simulink model "MASs_cp"  (R2015b)
settings: Solver=ode45  SolverMode=SingleTasking  StartTime=0.0  StopTime=10000  RelTol=1e-3
model workspace (MAT data in the model file):
  B = 3.17
  Cb = 0.251
  Izz = 1
  L = 9.8
  d = 0.71
  m = 5540
undefined symbols (not defined in the file or in its folder): magnitude
libraries: simulink x10
(part 1 of 2)
settings Model: Creator=Administrator  LastModifiedBy=Administrator
settings OptimizationCC: DefaultParameterBehavior=Inlined  UseFloatMulNetSlope=on  InlineInvariantSignals=on  PassReuseOutputArgsAs=Individual arguments  ZeroExternalMemoryAtStartup=off  ZeroInternalMemoryAtStartup=off  NoFixptDivByZeroProtection=on  EfficientFloat2IntCast=on  OptimizeModelRefInitCode=on  LifeSpan=1
settings HardwareCC: ProdBitPerPointer=32  ProdLargestAtomicInteger=Long  ProdLargestAtomicFloat=Double  ProdWordSize=32  ProdHWDeviceType=NXP->Cortex-M4
settings RTWCC: SystemTargetFile=ert.tlc  TemplateMakefile=ert_default_tmf  Description=Embedded Coder  GenerateReport=on  IncludeHyperlinkInReport=on  LaunchReport=on  GenerateTraceInfo=on  GenerateTraceReport=on  GenerateTraceReportSl=on  GenerateTraceReportSf=on  GenerateTraceReportEml=on  GenerateCodeMetricsReport=on
settings CodeAppCC: ForceParamTrailComments=on  IgnoreCustomStorageClasses=off  SimulinkDataObjDesc=on  CustomSymbolStrGlobalVar=rt$N$M  CustomSymbolStrType=$N$M  CustomSymbolStrFcn=$N$M$F  CustomSymbolStrMacro=$N$M  InsertBlockDesc=on
settings ERTTargetCC: GenerateSampleERTMain=on  IncludeMdlTerminateFcn=off  CombineSignalStateStructs=on  SupportNonFinite=off  SupportContinuousTime=on  InlinedParameterPlacement=NonHierarchical  ERTCustomFileTemplate=example_file_process.tlc  ERTFilePackagingFormat=CompactWithDataFile

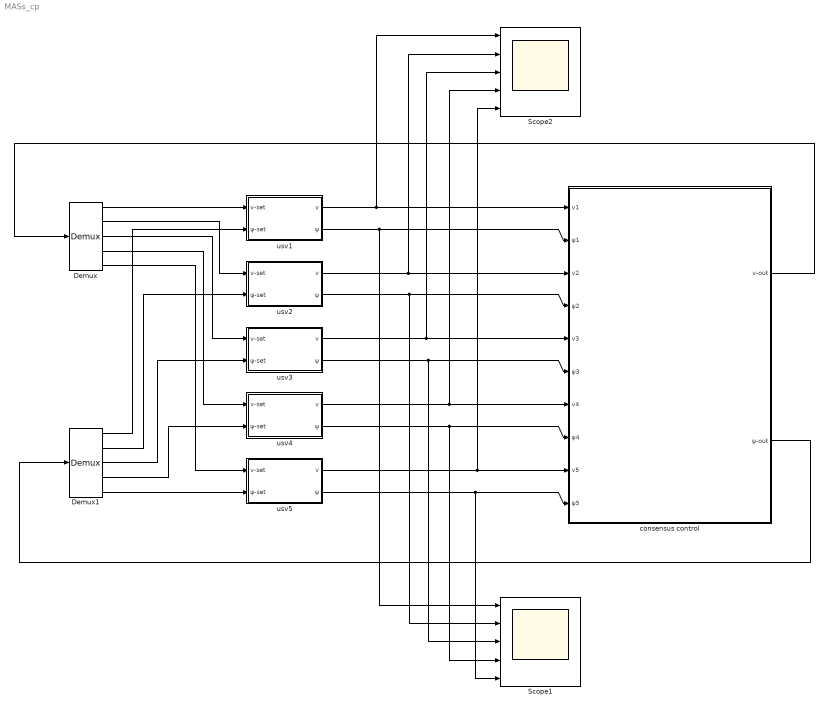
== system MASs_cp ==
  Demux : Demux  Outputs=5
  Demux1 : Demux  Outputs=5
  Scope1 : Scope  NumInputPorts=5
  Scope2 : Scope  NumInputPorts=5
  consensus control : Subsystem
  usv1 : Subsystem
  usv2 : Subsystem
  usv3 : Subsystem
  usv4 : Subsystem
  usv5 : Subsystem
  wires:
  usv1/2(ψ) -> Scope1/1, consensus control/2(ψ1)
  usv2/2(ψ) -> Scope1/2, consensus control/4(ψ2)
  usv3/2(ψ) -> Scope1/3, consensus control/6(ψ3)
  usv4/2(ψ) -> Scope1/4, consensus control/8(ψ4)
  usv5/2(ψ) -> Scope1/5, consensus control/10(ψ5)
  Demux/1 -> usv1/1(v-set)
  Demux/2 -> usv2/1(v-set)
  Demux/3 -> usv3/1(v-set)
  Demux/4 -> usv4/1(v-set)
  Demux/5 -> usv5/1(v-set)
  Demux1/2 -> usv2/2(ψ-set)
  Demux1/3 -> usv3/2(ψ-set)
  Demux1/4 -> usv4/2(ψ-set)
  Demux1/5 -> usv5/2(ψ-set)
  Demux1/1 -> usv1/2(ψ-set)
  usv1/1(v) -> Scope2/1, consensus control/1(v1)
  usv2/1(v) -> Scope2/2, consensus control/3(v2)
  usv3/1(v) -> Scope2/3, consensus control/5(v3)
  usv4/1(v) -> Scope2/4, consensus control/7(v4)
  usv5/1(v) -> Scope2/5, consensus control/9(v5)
  consensus control/2(ψ-out) -> Demux1/1
  consensus control/1(v-out) -> Demux/1

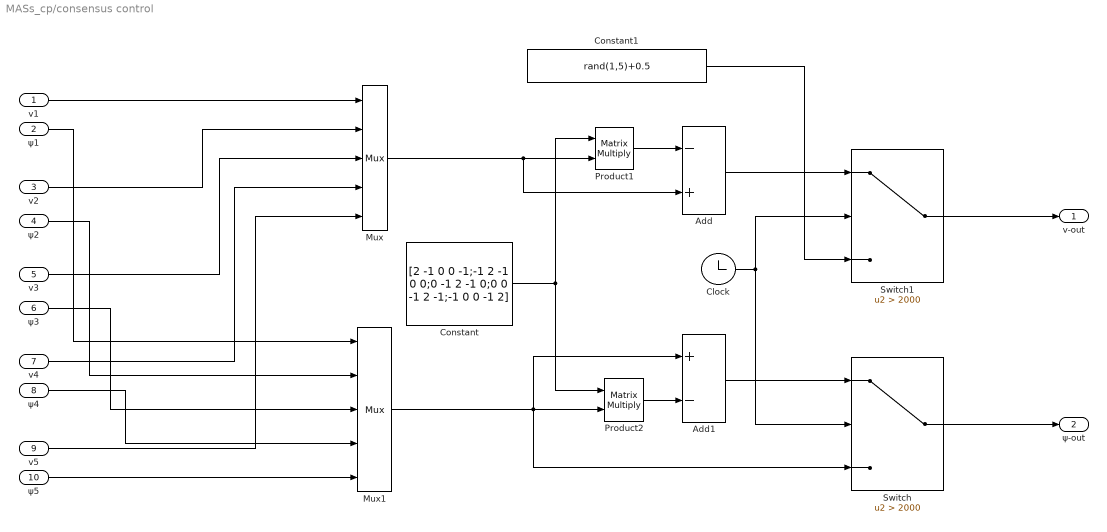
== system MASs_cp/consensus control ==
  v1 : Inport
  ψ1 : Inport  Port=2
  v2 : Inport  Port=3
  ψ2 : Inport  Port=4
  v3 : Inport  Port=5
  ψ3 : Inport  Port=6
  v4 : Inport  Port=7
  ψ4 : Inport  Port=8
  v5 : Inport  Port=9
  ψ5 : Inport  Port=10
  Add : Sum  Inputs=-+
  Add1 : Sum  Inputs=+-
  Clock : Clock
  Constant : Constant  Value=[2 -1 0 0 -1;-1 2 -1 0 0;0 -1 2 -1 0;0 0 -1 2 -1;-1 0 0 -1 2]  VectorParams1D=off
  Constant1 : Constant  Value=rand(1,5)+0.5
  Mux : Mux  Inputs=5
  Mux1 : Mux  Inputs=5
  Product1 : Product  Multiplication=Matrix(*)
  Product2 : Product  Multiplication=Matrix(*)
  Switch : Switch  Criteria=u2 > Threshold  Threshold=2000
  Switch1 : Switch  Criteria=u2 > Threshold  Threshold=2000
  v-out : Outport
  ψ-out : Outport  Port=2
  wires:
  Mux/1 -> Add/2, Product1/2
  Add/1 -> Switch1/1
  Product1/1 -> Add/1
  v4/1 -> Mux/4
  v5/1 -> Mux/5
  Mux1/1 -> Switch/3, Add1/1, Product2/2
  Product2/1 -> Add1/2
  ψ4/1 -> Mux1/4
  ψ1/1 -> Mux1/1
  ψ2/1 -> Mux1/2
  ψ3/1 -> Mux1/3
  ψ5/1 -> Mux1/5
  Add1/1 -> Switch/1
  v3/1 -> Mux/3
  v2/1 -> Mux/2
  Constant/1 -> Product2/1, Product1/1
  v1/1 -> Mux/1
  Clock/1 -> Switch/2, Switch1/2
  Switch/1 -> ψ-out/1
  Constant1/1 -> Switch1/3
  Switch1/1 -> v-out/1

== system MASs_cp/usv1 ==
  v-set : Inport
  ψ-set : Inport  Port=2
  Scope : Scope  NumInputPorts=3
  Scope1 : Scope  NumInputPorts=3
  To Workspace : ToWorkspace  VariableName=x1  SampleTime=-1
  To Workspace1 : ToWorkspace  VariableName=y1  SampleTime=-1
  USV : Subsystem
  direction-PID : Subsystem
  speed-PID : Subsystem
  v : Outport
  ψ : Outport  Port=2
  wires:
  speed-PID/1(output) -> USV/1(n)
  USV/6(ψ) -> Scope1/3, ψ/1, direction-PID/2(feedback)
  USV/3(r) -> Scope/3
  direction-PID/1(output) -> USV/2(δ)
  v-set/1 -> speed-PID/2(set)
  USV/2(v) -> Scope/2
  ψ-set/1 -> direction-PID/1(set)
  USV/5(y) -> To Workspace1/1, Scope1/2
  USV/4(x) -> To Workspace/1, Scope1/1
  USV/1(u) -> v/1, speed-PID/1(feedback), Scope/1

== system MASs_cp/usv2 ==
  v-set : Inport
  ψ-set : Inport  Port=2
  Scope : Scope  NumInputPorts=3
  Scope1 : Scope  NumInputPorts=3
  To Workspace : ToWorkspace  VariableName=x2  SampleTime=-1
  To Workspace1 : ToWorkspace  VariableName=y2  SampleTime=-1
  USV : Subsystem
  direction-PID : Subsystem
  speed-PID : Subsystem
  v : Outport
  ψ : Outport  Port=2
  wires:
  speed-PID/1(output) -> USV/1(n)
  USV/6(ψ) -> Scope1/3, ψ/1, direction-PID/2(feedback)
  USV/3(r) -> Scope/3
  direction-PID/1(output) -> USV/2(δ)
  v-set/1 -> speed-PID/2(set)
  USV/2(v) -> Scope/2
  ψ-set/1 -> direction-PID/1(set)
  USV/5(y) -> To Workspace1/1, Scope1/2
  USV/4(x) -> To Workspace/1, Scope1/1
  USV/1(u) -> speed-PID/1(feedback), v/1, Scope/1

== system MASs_cp/usv3 ==
  v-set : Inport
  ψ-set : Inport  Port=2
  Scope : Scope  NumInputPorts=3
  Scope1 : Scope  NumInputPorts=3
  To Workspace : ToWorkspace  VariableName=x3  SampleTime=-1
  To Workspace1 : ToWorkspace  VariableName=y3  SampleTime=-1
  USV : Subsystem
  direction-PID1 : Subsystem
  speed-PID : Subsystem
  v : Outport
  ψ : Outport  Port=2
  wires:
  speed-PID/1(output) -> USV/1(n)
  USV/6(ψ) -> Scope1/3, direction-PID1/2(feedback), ψ/1
  USV/3(r) -> Scope/3
  direction-PID1/1(output) -> USV/2(δ)
  v-set/1 -> speed-PID/2(set)
  USV/2(v) -> Scope/2
  ψ-set/1 -> direction-PID1/1(set)
  USV/5(y) -> To Workspace1/1, Scope1/2
  USV/4(x) -> To Workspace/1, Scope1/1
  USV/1(u) -> speed-PID/1(feedback), v/1, Scope/1

== system MASs_cp/usv4 ==
  v-set : Inport
  ψ-set : Inport  Port=2
  Scope : Scope  NumInputPorts=3
  Scope1 : Scope  NumInputPorts=3
  To Workspace : ToWorkspace  VariableName=x4  SampleTime=-1
  To Workspace1 : ToWorkspace  VariableName=y4  SampleTime=-1
  USV : Subsystem
  direction-PID : Subsystem
  speed-PID : Subsystem
  v : Outport
  ψ : Outport  Port=2
  wires:
  speed-PID/1(output) -> USV/1(n)
  USV/6(ψ) -> Scope1/3, direction-PID/2(feedback), ψ/1
  USV/3(r) -> Scope/3
  direction-PID/1(output) -> USV/2(δ)
  v-set/1 -> speed-PID/2(set)
  USV/2(v) -> Scope/2
  ψ-set/1 -> direction-PID/1(set)
  USV/5(y) -> To Workspace1/1, Scope1/2
  USV/4(x) -> To Workspace/1, Scope1/1
  USV/1(u) -> speed-PID/1(feedback), v/1, Scope/1

== system MASs_cp/usv5 ==
  v-set : Inport
  ψ-set : Inport  Port=2
  Scope : Scope  NumInputPorts=3
  Scope1 : Scope  NumInputPorts=3
  To Workspace : ToWorkspace  VariableName=x5  SampleTime=-1
  To Workspace1 : ToWorkspace  VariableName=y5  SampleTime=-1
  USV : Subsystem
  direction-PID : Subsystem
  speed-PID : Subsystem
  v : Outport
  ψ : Outport  Port=2
  wires:
  speed-PID/1(output) -> USV/1(n)
  USV/6(ψ) -> Scope1/3, direction-PID/2(feedback), ψ/1
  USV/3(r) -> Scope/3
  direction-PID/1(output) -> USV/2(δ)
  v-set/1 -> speed-PID/2(set)
  USV/2(v) -> Scope/2
  ψ-set/1 -> direction-PID/1(set)
  USV/5(y) -> To Workspace1/1, Scope1/2
  USV/4(x) -> To Workspace/1, Scope1/1
  USV/1(u) -> speed-PID/1(feedback), v/1, Scope/1

== system MASs_cp/usv1/USV ==
  n : Inport
  δ : Inport  Port=2
  F model : Subsystem
  M model : Subsystem
  motion model : Subsystem
  u : Outport
  v : Outport  Port=2
  r : Outport  Port=3
  x : Outport  Port=4
  y : Outport  Port=5
  ψ : Outport  Port=6
  wires:
  M model/5(Jzz) -> motion model/8(Jzz)
  M model/3(my) -> motion model/6(my)
  M model/1(m) -> motion model/4(m)
  F model/2(Y) -> motion model/2(Y)
  n/1 -> F model/1(n)
  δ/1 -> F model/2(δ)
  F model/1(X) -> motion model/1(X)
  motion model/1(u) -> u/1, F model/3(u)  "u"
  motion model/3(r) -> r/1, F model/5(r)  "r"
  motion model/2(v) -> v/1, F model/4(v)  "v"
  motion model/6(ψ) -> ψ/1  "ψ"
  F model/3(N) -> motion model/3(N)
  M model/2(mx) -> motion model/5(mx)
  M model/4(Izz) -> motion model/7(Izz)
  motion model/4(x) -> x/1  "x"
  motion model/5(y) -> y/1  "y"

== system MASs_cp/usv1/direction-PID ==
  set : Inport
  feedback : Inport  Port=2
  Gain : Gain  Gain=-1
  PID Controller : simulink/Continuous/PID Controller  Controller=PID  TimeDomain=Continuous-time  SampleTime=-1  IntegratorMethod=Forward Euler  FilterMethod=Forward Euler  Form=Parallel  UseFilter=on  ControllerParametersSource=internal  P=3  I=0  D=0  N=5.45397025421619  InitialConditionSource=internal  InitialConditionForIntegrator=0  InitialConditionForFilter=0  ExternalReset=none  LimitOutput=on  UpperSaturationLimit=50  LowerSaturationLimit=-50  LinearizeAsGain=on  AntiWindupMode=none  Kb=1  TrackingMode=off  Kt=1  PParamMin=[]  PParamMax=[]  IParamMin=[]  IParamMax=[]  DParamMin=[]  DParamMax=[]  NParamMin=[]  NParamMax=[]  KbParamMin=[]  KbParamMax=[]  KtParamMin=[]  KtParamMax=[]  POutMin=[]  POutMax=[]  IOutMin=[]  IOutMax=[]  DOutMin=[]  DOutMax=[]  NOutMin=[]  NOutMax=[]  KbOutMin=[]  KbOutMax=[]  KtOutMin=[]  KtOutMax=[]  IntegratorOutMin=[]  IntegratorOutMax=[]  FilterOutMin=[]  FilterOutMax=[]  SumOutMin=[]  SumOutMax=[]  SumI1OutMin=[]  SumI1OutMax=[]  SumI2OutMin=[]  SumI2OutMax=[]  SumI3OutMin=[]  SumI3OutMax=[]  SumDOutMin=[]  SumDOutMax=[]  SaturationOutMin=[]  SaturationOutMax=[]  IntegratorContinuousStateAttributes=''  IntegratorStateMustResolveToSignalObject=off  IntegratorRTWStateStorageClass=Auto  FilterContinuousStateAttributes=''  FilterStateMustResolveToSignalObject=off  FilterRTWStateStorageClass=Auto  DifferentiatorICPrevScaledInput=0  DifferentiatorOutMin=[]  DifferentiatorOutMax=[]
  Scope2 : Scope  NumInputPorts=3
  Sum : Sum  Inputs=|+-
  output : Outport
  wires:
  PID Controller/1 -> Gain/1, Scope2/3
  Sum/1 -> PID Controller/1
  set/1 -> Scope2/1, Sum/1
  feedback/1 -> Scope2/2, Sum/2
  Gain/1 -> output/1

== system MASs_cp/usv1/speed-PID ==
  feedback : Inport
  set : Inport  Port=2
  PID Controller : simulink/Continuous/PID Controller  Controller=PID  TimeDomain=Continuous-time  SampleTime=-1  IntegratorMethod=Forward Euler  FilterMethod=Forward Euler  Form=Parallel  UseFilter=on  ControllerParametersSource=internal  P=500  I=2  D=0  N=5.45397025421619  InitialConditionSource=internal  InitialConditionForIntegrator=0  InitialConditionForFilter=0  ExternalReset=none  LimitOutput=on  UpperSaturationLimit=2000  LowerSaturationLimit=0  LinearizeAsGain=on  AntiWindupMode=none  Kb=1  TrackingMode=off  Kt=1  PParamMin=[]  PParamMax=[]  IParamMin=[]  IParamMax=[]  DParamMin=[]  DParamMax=[]  NParamMin=[]  NParamMax=[]  KbParamMin=[]  KbParamMax=[]  KtParamMin=[]  KtParamMax=[]  POutMin=[]  POutMax=[]  IOutMin=[]  IOutMax=[]  DOutMin=[]  DOutMax=[]  NOutMin=[]  NOutMax=[]  KbOutMin=[]  KbOutMax=[]  KtOutMin=[]  KtOutMax=[]  IntegratorOutMin=[]  IntegratorOutMax=[]  FilterOutMin=[]  FilterOutMax=[]  SumOutMin=[]  SumOutMax=[]  SumI1OutMin=[]  SumI1OutMax=[]  SumI2OutMin=[]  SumI2OutMax=[]  SumI3OutMin=[]  SumI3OutMax=[]  SumDOutMin=[]  SumDOutMax=[]  SaturationOutMin=[]  SaturationOutMax=[]  IntegratorContinuousStateAttributes=''  IntegratorStateMustResolveToSignalObject=off  IntegratorRTWStateStorageClass=Auto  FilterContinuousStateAttributes=''  FilterStateMustResolveToSignalObject=off  FilterRTWStateStorageClass=Auto  DifferentiatorICPrevScaledInput=0  DifferentiatorOutMin=[]  DifferentiatorOutMax=[]
  Scope3 : Scope  NumInputPorts=3
  Sum1 : Sum  Inputs=|+-
  output : Outport
  wires:
  set/1 -> Sum1/1, Scope3/1
  PID Controller/1 -> output/1, Scope3/3
  Sum1/1 -> PID Controller/1
  feedback/1 -> Sum1/2, Scope3/2

== system MASs_cp/usv2/USV ==
  n : Inport
  δ : Inport  Port=2
  F model : Subsystem
  M model : Subsystem
  motion model : Subsystem
  u : Outport
  v : Outport  Port=2
  r : Outport  Port=3
  x : Outport  Port=4
  y : Outport  Port=5
  ψ : Outport  Port=6
  wires:
  M model/5(Jzz) -> motion model/8(Jzz)
  M model/3(my) -> motion model/6(my)
  M model/1(m) -> motion model/4(m)
  F model/2(Y) -> motion model/2(Y)
  n/1 -> F model/1(n)
  δ/1 -> F model/2(δ)
  F model/1(X) -> motion model/1(X)
  motion model/1(u) -> u/1, F model/3(u)  "u"
  motion model/3(r) -> r/1, F model/5(r)  "r"
  motion model/2(v) -> v/1, F model/4(v)  "v"
  motion model/6(ψ) -> ψ/1  "ψ"
  F model/3(N) -> motion model/3(N)
  M model/2(mx) -> motion model/5(mx)
  M model/4(Izz) -> motion model/7(Izz)
  motion model/4(x) -> x/1  "x"
  motion model/5(y) -> y/1  "y"

== system MASs_cp/usv2/direction-PID ==
  set : Inport
  feedback : Inport  Port=2
  Gain : Gain  Gain=-1
  PID Controller : simulink/Continuous/PID Controller  Controller=PID  TimeDomain=Continuous-time  SampleTime=-1  IntegratorMethod=Forward Euler  FilterMethod=Forward Euler  Form=Parallel  UseFilter=on  ControllerParametersSource=internal  P=3  I=0  D=0  N=5.45397025421619  InitialConditionSource=internal  InitialConditionForIntegrator=0  InitialConditionForFilter=0  ExternalReset=none  LimitOutput=on  UpperSaturationLimit=50  LowerSaturationLimit=-50  LinearizeAsGain=on  AntiWindupMode=none  Kb=1  TrackingMode=off  Kt=1  PParamMin=[]  PParamMax=[]  IParamMin=[]  IParamMax=[]  DParamMin=[]  DParamMax=[]  NParamMin=[]  NParamMax=[]  KbParamMin=[]  KbParamMax=[]  KtParamMin=[]  KtParamMax=[]  POutMin=[]  POutMax=[]  IOutMin=[]  IOutMax=[]  DOutMin=[]  DOutMax=[]  NOutMin=[]  NOutMax=[]  KbOutMin=[]  KbOutMax=[]  KtOutMin=[]  KtOutMax=[]  IntegratorOutMin=[]  IntegratorOutMax=[]  FilterOutMin=[]  FilterOutMax=[]  SumOutMin=[]  SumOutMax=[]  SumI1OutMin=[]  SumI1OutMax=[]  SumI2OutMin=[]  SumI2OutMax=[]  SumI3OutMin=[]  SumI3OutMax=[]  SumDOutMin=[]  SumDOutMax=[]  SaturationOutMin=[]  SaturationOutMax=[]  IntegratorContinuousStateAttributes=''  IntegratorStateMustResolveToSignalObject=off  IntegratorRTWStateStorageClass=Auto  FilterContinuousStateAttributes=''  FilterStateMustResolveToSignalObject=off  FilterRTWStateStorageClass=Auto  DifferentiatorICPrevScaledInput=0  DifferentiatorOutMin=[]  DifferentiatorOutMax=[]
  Scope2 : Scope  NumInputPorts=3
  Sum : Sum  Inputs=|+-
  output : Outport
  wires:
  PID Controller/1 -> Gain/1, Scope2/3
  Sum/1 -> PID Controller/1
  set/1 -> Scope2/1, Sum/1
  feedback/1 -> Scope2/2, Sum/2
  Gain/1 -> output/1

== system MASs_cp/usv2/speed-PID ==
  feedback : Inport
  set : Inport  Port=2
  PID Controller : simulink/Continuous/PID Controller  Controller=PID  TimeDomain=Continuous-time  SampleTime=-1  IntegratorMethod=Forward Euler  FilterMethod=Forward Euler  Form=Parallel  UseFilter=on  ControllerParametersSource=internal  P=500  I=2  D=0  N=5.45397025421619  InitialConditionSource=internal  InitialConditionForIntegrator=0  InitialConditionForFilter=0  ExternalReset=none  LimitOutput=on  UpperSaturationLimit=2000  LowerSaturationLimit=0  LinearizeAsGain=on  AntiWindupMode=none  Kb=1  TrackingMode=off  Kt=1  PParamMin=[]  PParamMax=[]  IParamMin=[]  IParamMax=[]  DParamMin=[]  DParamMax=[]  NParamMin=[]  NParamMax=[]  KbParamMin=[]  KbParamMax=[]  KtParamMin=[]  KtParamMax=[]  POutMin=[]  POutMax=[]  IOutMin=[]  IOutMax=[]  DOutMin=[]  DOutMax=[]  NOutMin=[]  NOutMax=[]  KbOutMin=[]  KbOutMax=[]  KtOutMin=[]  KtOutMax=[]  IntegratorOutMin=[]  IntegratorOutMax=[]  FilterOutMin=[]  FilterOutMax=[]  SumOutMin=[]  SumOutMax=[]  SumI1OutMin=[]  SumI1OutMax=[]  SumI2OutMin=[]  SumI2OutMax=[]  SumI3OutMin=[]  SumI3OutMax=[]  SumDOutMin=[]  SumDOutMax=[]  SaturationOutMin=[]  SaturationOutMax=[]  IntegratorContinuousStateAttributes=''  IntegratorStateMustResolveToSignalObject=off  IntegratorRTWStateStorageClass=Auto  FilterContinuousStateAttributes=''  FilterStateMustResolveToSignalObject=off  FilterRTWStateStorageClass=Auto  DifferentiatorICPrevScaledInput=0  DifferentiatorOutMin=[]  DifferentiatorOutMax=[]
  Scope3 : Scope  NumInputPorts=3
  Sum1 : Sum  Inputs=|+-
  output : Outport
  wires:
  set/1 -> Sum1/1, Scope3/1
  PID Controller/1 -> output/1, Scope3/3
  Sum1/1 -> PID Controller/1
  feedback/1 -> Sum1/2, Scope3/2

== system MASs_cp/usv3/USV ==
  n : Inport
  δ : Inport  Port=2
  F model : Subsystem
  M model : Subsystem
  motion model : Subsystem
  u : Outport
  v : Outport  Port=2
  r : Outport  Port=3
  x : Outport  Port=4
  y : Outport  Port=5
  ψ : Outport  Port=6
  wires:
  M model/5(Jzz) -> motion model/8(Jzz)
  M model/3(my) -> motion model/6(my)
  M model/1(m) -> motion model/4(m)
  F model/2(Y) -> motion model/2(Y)
  n/1 -> F model/1(n)
  δ/1 -> F model/2(δ)
  F model/1(X) -> motion model/1(X)
  motion model/1(u) -> u/1, F model/3(u)  "u"
  motion model/3(r) -> r/1, F model/5(r)  "r"
  motion model/2(v) -> v/1, F model/4(v)  "v"
  motion model/6(ψ) -> ψ/1  "ψ"
  F model/3(N) -> motion model/3(N)
  M model/2(mx) -> motion model/5(mx)
  M model/4(Izz) -> motion model/7(Izz)
  motion model/4(x) -> x/1  "x"
  motion model/5(y) -> y/1  "y"

== system MASs_cp/usv3/direction-PID1 ==
  set : Inport
  feedback : Inport  Port=2
  Gain : Gain  Gain=-1
  PID Controller : simulink/Continuous/PID Controller  Controller=PID  TimeDomain=Continuous-time  SampleTime=-1  IntegratorMethod=Forward Euler  FilterMethod=Forward Euler  Form=Parallel  UseFilter=on  ControllerParametersSource=internal  P=3  I=0  D=0  N=5.45397025421619  InitialConditionSource=internal  InitialConditionForIntegrator=0  InitialConditionForFilter=0  ExternalReset=none  LimitOutput=on  UpperSaturationLimit=50  LowerSaturationLimit=-50  LinearizeAsGain=on  AntiWindupMode=none  Kb=1  TrackingMode=off  Kt=1  PParamMin=[]  PParamMax=[]  IParamMin=[]  IParamMax=[]  DParamMin=[]  DParamMax=[]  NParamMin=[]  NParamMax=[]  KbParamMin=[]  KbParamMax=[]  KtParamMin=[]  KtParamMax=[]  POutMin=[]  POutMax=[]  IOutMin=[]  IOutMax=[]  DOutMin=[]  DOutMax=[]  NOutMin=[]  NOutMax=[]  KbOutMin=[]  KbOutMax=[]  KtOutMin=[]  KtOutMax=[]  IntegratorOutMin=[]  IntegratorOutMax=[]  FilterOutMin=[]  FilterOutMax=[]  SumOutMin=[]  SumOutMax=[]  SumI1OutMin=[]  SumI1OutMax=[]  SumI2OutMin=[]  SumI2OutMax=[]  SumI3OutMin=[]  SumI3OutMax=[]  SumDOutMin=[]  SumDOutMax=[]  SaturationOutMin=[]  SaturationOutMax=[]  IntegratorContinuousStateAttributes=''  IntegratorStateMustResolveToSignalObject=off  IntegratorRTWStateStorageClass=Auto  FilterContinuousStateAttributes=''  FilterStateMustResolveToSignalObject=off  FilterRTWStateStorageClass=Auto  DifferentiatorICPrevScaledInput=0  DifferentiatorOutMin=[]  DifferentiatorOutMax=[]
  Scope2 : Scope  NumInputPorts=3
  Sum : Sum  Inputs=|+-
  output : Outport
  wires:
  PID Controller/1 -> Gain/1, Scope2/3
  Sum/1 -> PID Controller/1
  set/1 -> Scope2/1, Sum/1
  feedback/1 -> Scope2/2, Sum/2
  Gain/1 -> output/1

== system MASs_cp/usv3/speed-PID ==
  feedback : Inport
  set : Inport  Port=2
  PID Controller : simulink/Continuous/PID Controller  Controller=PID  TimeDomain=Continuous-time  SampleTime=-1  IntegratorMethod=Forward Euler  FilterMethod=Forward Euler  Form=Parallel  UseFilter=on  ControllerParametersSource=internal  P=500  I=2  D=0  N=5.45397025421619  InitialConditionSource=internal  InitialConditionForIntegrator=0  InitialConditionForFilter=0  ExternalReset=none  LimitOutput=on  UpperSaturationLimit=2000  LowerSaturationLimit=0  LinearizeAsGain=on  AntiWindupMode=none  Kb=1  TrackingMode=off  Kt=1  PParamMin=[]  PParamMax=[]  IParamMin=[]  IParamMax=[]  DParamMin=[]  DParamMax=[]  NParamMin=[]  NParamMax=[]  KbParamMin=[]  KbParamMax=[]  KtParamMin=[]  KtParamMax=[]  POutMin=[]  POutMax=[]  IOutMin=[]  IOutMax=[]  DOutMin=[]  DOutMax=[]  NOutMin=[]  NOutMax=[]  KbOutMin=[]  KbOutMax=[]  KtOutMin=[]  KtOutMax=[]  IntegratorOutMin=[]  IntegratorOutMax=[]  FilterOutMin=[]  FilterOutMax=[]  SumOutMin=[]  SumOutMax=[]  SumI1OutMin=[]  SumI1OutMax=[]  SumI2OutMin=[]  SumI2OutMax=[]  SumI3OutMin=[]  SumI3OutMax=[]  SumDOutMin=[]  SumDOutMax=[]  SaturationOutMin=[]  SaturationOutMax=[]  IntegratorContinuousStateAttributes=''  IntegratorStateMustResolveToSignalObject=off  IntegratorRTWStateStorageClass=Auto  FilterContinuousStateAttributes=''  FilterStateMustResolveToSignalObject=off  FilterRTWStateStorageClass=Auto  DifferentiatorICPrevScaledInput=0  DifferentiatorOutMin=[]  DifferentiatorOutMax=[]
  Scope3 : Scope  NumInputPorts=3
  Sum1 : Sum  Inputs=|+-
  output : Outport
  wires:
  set/1 -> Sum1/1, Scope3/1
  PID Controller/1 -> output/1, Scope3/3
  Sum1/1 -> PID Controller/1
  feedback/1 -> Sum1/2, Scope3/2

== system MASs_cp/usv4/USV ==
  n : Inport
  δ : Inport  Port=2
  F model : Subsystem
  M model : Subsystem
  motion model : Subsystem
  u : Outport
  v : Outport  Port=2
  r : Outport  Port=3
  x : Outport  Port=4
  y : Outport  Port=5
  ψ : Outport  Port=6
  wires:
  M model/5(Jzz) -> motion model/8(Jzz)
  M model/3(my) -> motion model/6(my)
  M model/1(m) -> motion model/4(m)
  F model/2(Y) -> motion model/2(Y)
  n/1 -> F model/1(n)
  δ/1 -> F model/2(δ)
  F model/1(X) -> motion model/1(X)
  motion model/1(u) -> u/1, F model/3(u)  "u"
  motion model/3(r) -> r/1, F model/5(r)  "r"
  motion model/2(v) -> v/1, F model/4(v)  "v"
  motion model/6(ψ) -> ψ/1  "ψ"
  F model/3(N) -> motion model/3(N)
  M model/2(mx) -> motion model/5(mx)
  M model/4(Izz) -> motion model/7(Izz)
  motion model/4(x) -> x/1  "x"
  motion model/5(y) -> y/1  "y"

== system MASs_cp/usv4/direction-PID ==
  set : Inport
  feedback : Inport  Port=2
  Gain : Gain  Gain=-1
  PID Controller : simulink/Continuous/PID Controller  Controller=PID  TimeDomain=Continuous-time  SampleTime=-1  IntegratorMethod=Forward Euler  FilterMethod=Forward Euler  Form=Parallel  UseFilter=on  ControllerParametersSource=internal  P=3  I=0  D=0  N=5.45397025421619  InitialConditionSource=internal  InitialConditionForIntegrator=0  InitialConditionForFilter=0  ExternalReset=none  LimitOutput=on  UpperSaturationLimit=50  LowerSaturationLimit=-50  LinearizeAsGain=on  AntiWindupMode=none  Kb=1  TrackingMode=off  Kt=1  PParamMin=[]  PParamMax=[]  IParamMin=[]  IParamMax=[]  DParamMin=[]  DParamMax=[]  NParamMin=[]  NParamMax=[]  KbParamMin=[]  KbParamMax=[]  KtParamMin=[]  KtParamMax=[]  POutMin=[]  POutMax=[]  IOutMin=[]  IOutMax=[]  DOutMin=[]  DOutMax=[]  NOutMin=[]  NOutMax=[]  KbOutMin=[]  KbOutMax=[]  KtOutMin=[]  KtOutMax=[]  IntegratorOutMin=[]  IntegratorOutMax=[]  FilterOutMin=[]  FilterOutMax=[]  SumOutMin=[]  SumOutMax=[]  SumI1OutMin=[]  SumI1OutMax=[]  SumI2OutMin=[]  SumI2OutMax=[]  SumI3OutMin=[]  SumI3OutMax=[]  SumDOutMin=[]  SumDOutMax=[]  SaturationOutMin=[]  SaturationOutMax=[]  IntegratorContinuousStateAttributes=''  IntegratorStateMustResolveToSignalObject=off  IntegratorRTWStateStorageClass=Auto  FilterContinuousStateAttributes=''  FilterStateMustResolveToSignalObject=off  FilterRTWStateStorageClass=Auto  DifferentiatorICPrevScaledInput=0  DifferentiatorOutMin=[]  DifferentiatorOutMax=[]
  Scope2 : Scope  NumInputPorts=3
  Sum : Sum  Inputs=|+-
  output : Outport
  wires:
  PID Controller/1 -> Gain/1, Scope2/3
  Sum/1 -> PID Controller/1
  set/1 -> Scope2/1, Sum/1
  feedback/1 -> Scope2/2, Sum/2
  Gain/1 -> output/1

== system MASs_cp/usv4/speed-PID ==
  feedback : Inport
  set : Inport  Port=2
  PID Controller : simulink/Continuous/PID Controller  Controller=PID  TimeDomain=Continuous-time  SampleTime=-1  IntegratorMethod=Forward Euler  FilterMethod=Forward Euler  Form=Parallel  UseFilter=on  ControllerParametersSource=internal  P=500  I=2  D=0  N=5.45397025421619  InitialConditionSource=internal  InitialConditionForIntegrator=0  InitialConditionForFilter=0  ExternalReset=none  LimitOutput=on  UpperSaturationLimit=2000  LowerSaturationLimit=0  LinearizeAsGain=on  AntiWindupMode=none  Kb=1  TrackingMode=off  Kt=1  PParamMin=[]  PParamMax=[]  IParamMin=[]  IParamMax=[]  DParamMin=[]  DParamMax=[]  NParamMin=[]  NParamMax=[]  KbParamMin=[]  KbParamMax=[]  KtParamMin=[]  KtParamMax=[]  POutMin=[]  POutMax=[]  IOutMin=[]  IOutMax=[]  DOutMin=[]  DOutMax=[]  NOutMin=[]  NOutMax=[]  KbOutMin=[]  KbOutMax=[]  KtOutMin=[]  KtOutMax=[]  IntegratorOutMin=[]  IntegratorOutMax=[]  FilterOutMin=[]  FilterOutMax=[]  SumOutMin=[]  SumOutMax=[]  SumI1OutMin=[]  SumI1OutMax=[]  SumI2OutMin=[]  SumI2OutMax=[]  SumI3OutMin=[]  SumI3OutMax=[]  SumDOutMin=[]  SumDOutMax=[]  SaturationOutMin=[]  SaturationOutMax=[]  IntegratorContinuousStateAttributes=''  IntegratorStateMustResolveToSignalObject=off  IntegratorRTWStateStorageClass=Auto  FilterContinuousStateAttributes=''  FilterStateMustResolveToSignalObject=off  FilterRTWStateStorageClass=Auto  DifferentiatorICPrevScaledInput=0  DifferentiatorOutMin=[]  DifferentiatorOutMax=[]
  Scope3 : Scope  NumInputPorts=3
  Sum1 : Sum  Inputs=|+-
  output : Outport
  wires:
  set/1 -> Sum1/1, Scope3/1
  PID Controller/1 -> output/1, Scope3/3
  Sum1/1 -> PID Controller/1
  feedback/1 -> Sum1/2, Scope3/2

== system MASs_cp/usv5/USV ==
  n : Inport
  δ : Inport  Port=2
  F model : Subsystem
  M model : Subsystem
  motion model : Subsystem
  u : Outport
  v : Outport  Port=2
  r : Outport  Port=3
  x : Outport  Port=4
  y : Outport  Port=5
  ψ : Outport  Port=6
  wires:
  M model/5(Jzz) -> motion model/8(Jzz)
  M model/3(my) -> motion model/6(my)
  M model/1(m) -> motion model/4(m)
  F model/2(Y) -> motion model/2(Y)
  n/1 -> F model/1(n)
  δ/1 -> F model/2(δ)
  F model/1(X) -> motion model/1(X)
  motion model/1(u) -> u/1, F model/3(u)  "u"
  motion model/3(r) -> r/1, F model/5(r)  "r"
  motion model/2(v) -> v/1, F model/4(v)  "v"
  motion model/6(ψ) -> ψ/1  "ψ"
  F model/3(N) -> motion model/3(N)
  M model/2(mx) -> motion model/5(mx)
  M model/4(Izz) -> motion model/7(Izz)
  motion model/4(x) -> x/1  "x"
  motion model/5(y) -> y/1  "y"

== system MASs_cp/usv5/direction-PID ==
  set : Inport
  feedback : Inport  Port=2
  Gain : Gain  Gain=-1
  PID Controller : simulink/Continuous/PID Controller  Controller=PID  TimeDomain=Continuous-time  SampleTime=-1  IntegratorMethod=Forward Euler  FilterMethod=Forward Euler  Form=Parallel  UseFilter=on  ControllerParametersSource=internal  P=3  I=0  D=0  N=5.45397025421619  InitialConditionSource=internal  InitialConditionForIntegrator=0  InitialConditionForFilter=0  ExternalReset=none  LimitOutput=on  UpperSaturationLimit=50  LowerSaturationLimit=-50  LinearizeAsGain=on  AntiWindupMode=none  Kb=1  TrackingMode=off  Kt=1  PParamMin=[]  PParamMax=[]  IParamMin=[]  IParamMax=[]  DParamMin=[]  DParamMax=[]  NParamMin=[]  NParamMax=[]  KbParamMin=[]  KbParamMax=[]  KtParamMin=[]  KtParamMax=[]  POutMin=[]  POutMax=[]  IOutMin=[]  IOutMax=[]  DOutMin=[]  DOutMax=[]  NOutMin=[]  NOutMax=[]  KbOutMin=[]  KbOutMax=[]  KtOutMin=[]  KtOutMax=[]  IntegratorOutMin=[]  IntegratorOutMax=[]  FilterOutMin=[]  FilterOutMax=[]  SumOutMin=[]  SumOutMax=[]  SumI1OutMin=[]  SumI1OutMax=[]  SumI2OutMin=[]  SumI2OutMax=[]  SumI3OutMin=[]  SumI3OutMax=[]  SumDOutMin=[]  SumDOutMax=[]  SaturationOutMin=[]  SaturationOutMax=[]  IntegratorContinuousStateAttributes=''  IntegratorStateMustResolveToSignalObject=off  IntegratorRTWStateStorageClass=Auto  FilterContinuousStateAttributes=''  FilterStateMustResolveToSignalObject=off  FilterRTWStateStorageClass=Auto  DifferentiatorICPrevScaledInput=0  DifferentiatorOutMin=[]  DifferentiatorOutMax=[]
  Scope2 : Scope  NumInputPorts=3
  Sum : Sum  Inputs=|+-
  output : Outport
  wires:
  PID Controller/1 -> Gain/1, Scope2/3
  Sum/1 -> PID Controller/1
  set/1 -> Scope2/1, Sum/1
  feedback/1 -> Scope2/2, Sum/2
  Gain/1 -> output/1

== system MASs_cp/usv5/speed-PID ==
  feedback : Inport
  set : Inport  Port=2
  PID Controller : simulink/Continuous/PID Controller  Controller=PID  TimeDomain=Continuous-time  SampleTime=-1  IntegratorMethod=Forward Euler  FilterMethod=Forward Euler  Form=Parallel  UseFilter=on  ControllerParametersSource=internal  P=500  I=2  D=0  N=5.45397025421619  InitialConditionSource=internal  InitialConditionForIntegrator=0  InitialConditionForFilter=0  ExternalReset=none  LimitOutput=on  UpperSaturationLimit=2000  LowerSaturationLimit=0  LinearizeAsGain=on  AntiWindupMode=none  Kb=1  TrackingMode=off  Kt=1  PParamMin=[]  PParamMax=[]  IParamMin=[]  IParamMax=[]  DParamMin=[]  DParamMax=[]  NParamMin=[]  NParamMax=[]  KbParamMin=[]  KbParamMax=[]  KtParamMin=[]  KtParamMax=[]  POutMin=[]  POutMax=[]  IOutMin=[]  IOutMax=[]  DOutMin=[]  DOutMax=[]  NOutMin=[]  NOutMax=[]  KbOutMin=[]  KbOutMax=[]  KtOutMin=[]  KtOutMax=[]  IntegratorOutMin=[]  IntegratorOutMax=[]  FilterOutMin=[]  FilterOutMax=[]  SumOutMin=[]  SumOutMax=[]  SumI1OutMin=[]  SumI1OutMax=[]  SumI2OutMin=[]  SumI2OutMax=[]  SumI3OutMin=[]  SumI3OutMax=[]  SumDOutMin=[]  SumDOutMax=[]  SaturationOutMin=[]  SaturationOutMax=[]  IntegratorContinuousStateAttributes=''  IntegratorStateMustResolveToSignalObject=off  IntegratorRTWStateStorageClass=Auto  FilterContinuousStateAttributes=''  FilterStateMustResolveToSignalObject=off  FilterRTWStateStorageClass=Auto  DifferentiatorICPrevScaledInput=0  DifferentiatorOutMin=[]  DifferentiatorOutMax=[]
  Scope3 : Scope  NumInputPorts=3
  Sum1 : Sum  Inputs=|+-
  output : Outport
  wires:
  set/1 -> Sum1/1, Scope3/1
  PID Controller/1 -> output/1, Scope3/3
  Sum1/1 -> PID Controller/1
  feedback/1 -> Sum1/2, Scope3/2

== system MASs_cp/usv1/USV/F model ==
  n : Inport
  δ : Inport  Port=2
  u : Inport  Port=3
  v : Inport  Port=4
  r : Inport  Port=5
  Add : Sum  Inputs=3
  Add1 : Sum  Inputs=3
  Add2 : Sum  Inputs=3
  P model : Subsystem
  S model : Subsystem
  W model : Subsystem
  X : Outport
  Y : Outport  Port=2
  N : Outport  Port=3
  wires:
  n/1 -> P model/1(n)
  δ/1 -> P model/2(δ)
  P model/1(Xp) -> Add/1
  W model/1(Xw) -> Add/2
  S model/1(Xs) -> Add/3
  P model/2(Yp) -> Add1/1
  W model/2(Yw) -> Add1/2
  S model/2(Ys) -> Add1/3
  P model/3(Np) -> Add2/1
  W model/3(Nw) -> Add2/2
  S model/3(Ns) -> Add2/3
  Add/1 -> X/1
  Add1/1 -> Y/1
  Add2/1 -> N/1
  u/1 -> S model/1(u), P model/3(u)
  v/1 -> S model/2(v), P model/4(v)
  r/1 -> S model/3(r)

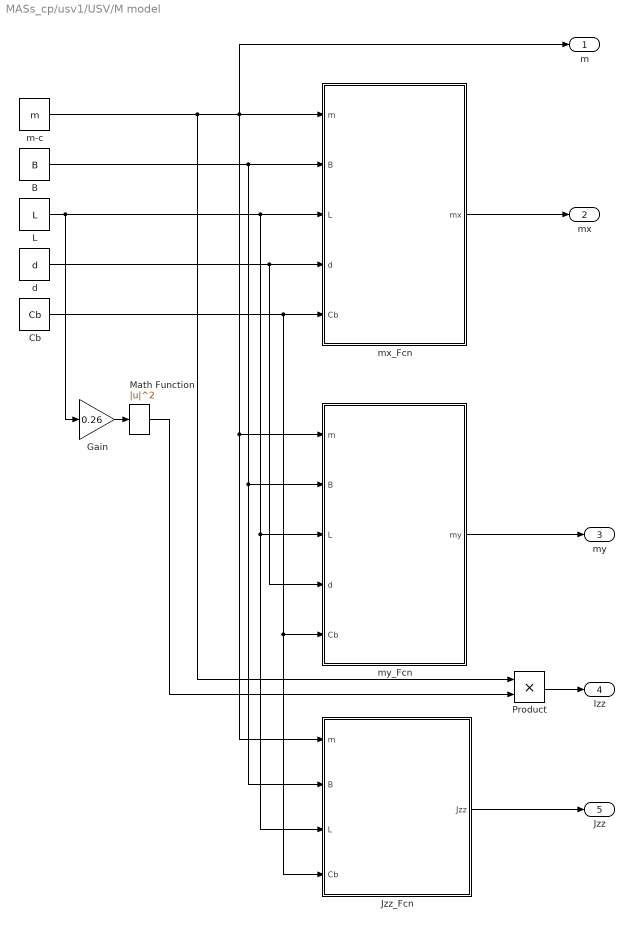
== system MASs_cp/usv1/USV/M model ==
  B : Constant  Value=B
  Cb : Constant  Value=Cb
  Gain : Gain  Gain=0.26
  Jzz_Fcn : MATLAB Function  TreatAsAtomicUnit=on
  L : Constant  Value=L
  Math Function : Math  Operator=magnitude^2  SaturateOnIntegerOverflow=on
  Product : Product
  d : Constant  Value=d
  m-c : Constant  Value=m
  mx_Fcn : MATLAB Function  TreatAsAtomicUnit=on
  my_Fcn : MATLAB Function  TreatAsAtomicUnit=on
  m : Outport
  mx : Outport  Port=2
  my : Outport  Port=3
  Izz : Outport  Port=4
  Jzz : Outport  Port=5
  wires:
  mx_Fcn/1(mx) -> mx/1
  d/1 -> my_Fcn/4(d), mx_Fcn/4(d)
  B/1 -> Jzz_Fcn/2(B), my_Fcn/2(B), mx_Fcn/2(B)
  my_Fcn/1(my) -> my/1
  Jzz_Fcn/1(Jzz) -> Jzz/1
  m-c/1 -> Product/1, m/1, Jzz_Fcn/1(m), my_Fcn/1(m), mx_Fcn/1(m)
  L/1 -> Gain/1, Jzz_Fcn/3(L), my_Fcn/3(L), mx_Fcn/3(L)
  Cb/1 -> Jzz_Fcn/4(Cb), my_Fcn/5(Cb), mx_Fcn/5(Cb)
  Gain/1 -> Math Function/1
  Product/1 -> Izz/1
  Math Function/1 -> Product/2

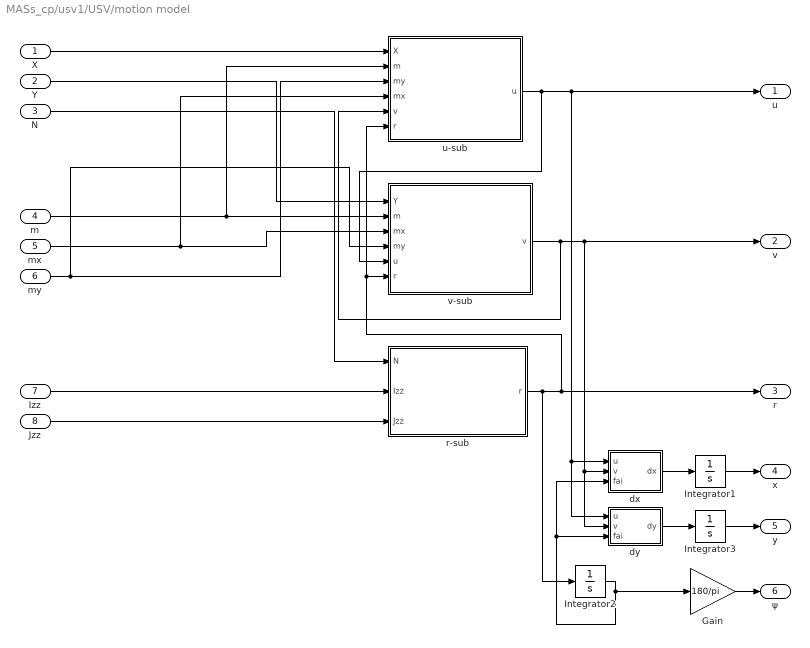
== system MASs_cp/usv1/USV/motion model ==
  X : Inport
  Y : Inport  Port=2
  N : Inport  Port=3
  m : Inport  Port=4
  mx : Inport  Port=5
  my : Inport  Port=6
  Izz : Inport  Port=7
  Jzz : Inport  Port=8
  Gain : Gain  Gain=180/pi
  Integrator1 : Integrator
  Integrator2 : Integrator  InitialCondition=rand()*pi-pi/2
  Integrator3 : Integrator
  dx : MATLAB Function  TreatAsAtomicUnit=on
  dy : MATLAB Function  TreatAsAtomicUnit=on
  r-sub : Subsystem
  u-sub : Subsystem
  v-sub : Subsystem
  u : Outport
  v : Outport  Port=2
  r : Outport  Port=3
  x : Outport  Port=4
  y : Outport  Port=5
  ψ : Outport  Port=6
  wires:
  m/1 -> v-sub/2(m), u-sub/2(m)
  Y/1 -> v-sub/1(Y)
  r-sub/1(r) -> r/1, u-sub/6(r), v-sub/6(r), Integrator2/1
  Izz/1 -> r-sub/2(Izz)
  N/1 -> r-sub/1(N)
  Jzz/1 -> r-sub/3(Jzz)
  X/1 -> u-sub/1(X)
  my/1 -> u-sub/3(my), v-sub/4(my)
  mx/1 -> u-sub/4(mx), v-sub/3(mx)
  v-sub/1(v) -> dy/2(v), dx/2(v), v/1, u-sub/5(v)
  u-sub/1(u) -> u/1, dy/1(u), dx/1(u), v-sub/5(u)
  dy/1(dy) -> Integrator3/1
  dx/1(dx) -> Integrator1/1
  Integrator3/1 -> y/1
  Integrator1/1 -> x/1
  Gain/1 -> ψ/1
  Integrator2/1 -> Gain/1, dy/3(fai), dx/3(fai)

== system MASs_cp/usv2/USV/F model ==
  n : Inport
  δ : Inport  Port=2
  u : Inport  Port=3
  v : Inport  Port=4
  r : Inport  Port=5
  Add : Sum  Inputs=3
  Add1 : Sum  Inputs=3
  Add2 : Sum  Inputs=3
  P model : Subsystem
  S model : Subsystem
  W model : Subsystem
  X : Outport
  Y : Outport  Port=2
  N : Outport  Port=3
  wires:
  n/1 -> P model/1(n)
  δ/1 -> P model/2(δ)
  P model/1(Xp) -> Add/1
  W model/1(Xw) -> Add/2
  S model/1(Xs) -> Add/3
  P model/2(Yp) -> Add1/1
  W model/2(Yw) -> Add1/2
  S model/2(Ys) -> Add1/3
  P model/3(Np) -> Add2/1
  W model/3(Nw) -> Add2/2
  S model/3(Ns) -> Add2/3
  Add/1 -> X/1
  Add1/1 -> Y/1
  Add2/1 -> N/1
  u/1 -> S model/1(u), P model/3(u)
  v/1 -> S model/2(v), P model/4(v)
  r/1 -> S model/3(r)

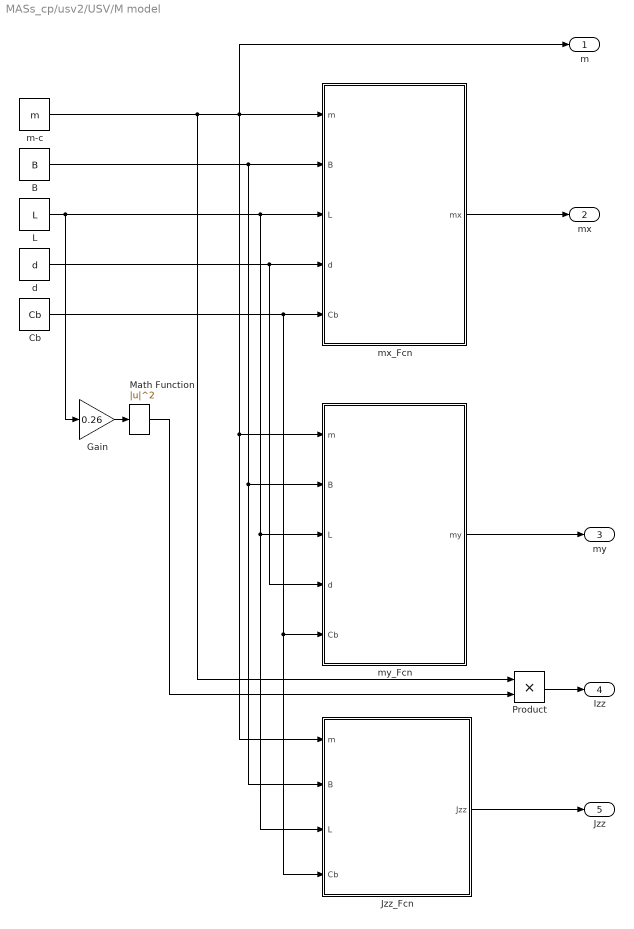
== system MASs_cp/usv2/USV/M model ==
  B : Constant  Value=B
  Cb : Constant  Value=Cb
  Gain : Gain  Gain=0.26
  Jzz_Fcn : MATLAB Function  TreatAsAtomicUnit=on
  L : Constant  Value=L
  Math Function : Math  Operator=magnitude^2  SaturateOnIntegerOverflow=on
  Product : Product
  d : Constant  Value=d
  m-c : Constant  Value=m
  mx_Fcn : MATLAB Function  TreatAsAtomicUnit=on
  my_Fcn : MATLAB Function  TreatAsAtomicUnit=on
  m : Outport
  mx : Outport  Port=2
  my : Outport  Port=3
  Izz : Outport  Port=4
  Jzz : Outport  Port=5
  wires:
  mx_Fcn/1(mx) -> mx/1
  d/1 -> my_Fcn/4(d), mx_Fcn/4(d)
  B/1 -> Jzz_Fcn/2(B), my_Fcn/2(B), mx_Fcn/2(B)
  my_Fcn/1(my) -> my/1
  Jzz_Fcn/1(Jzz) -> Jzz/1
  m-c/1 -> Product/1, m/1, Jzz_Fcn/1(m), my_Fcn/1(m), mx_Fcn/1(m)
  L/1 -> Gain/1, Jzz_Fcn/3(L), my_Fcn/3(L), mx_Fcn/3(L)
  Cb/1 -> Jzz_Fcn/4(Cb), my_Fcn/5(Cb), mx_Fcn/5(Cb)
  Gain/1 -> Math Function/1
  Product/1 -> Izz/1
  Math Function/1 -> Product/2

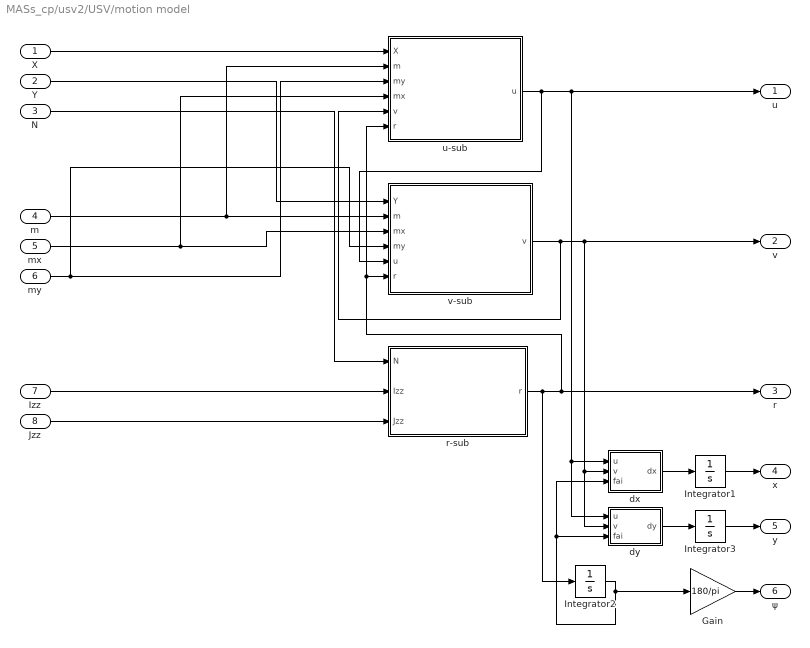
== system MASs_cp/usv2/USV/motion model ==
  X : Inport
  Y : Inport  Port=2
  N : Inport  Port=3
  m : Inport  Port=4
  mx : Inport  Port=5
  my : Inport  Port=6
  Izz : Inport  Port=7
  Jzz : Inport  Port=8
  Gain : Gain  Gain=180/pi
  Integrator1 : Integrator
  Integrator2 : Integrator  InitialCondition=rand()*pi-pi/2
  Integrator3 : Integrator
  dx : MATLAB Function  TreatAsAtomicUnit=on
  dy : MATLAB Function  TreatAsAtomicUnit=on
  r-sub : Subsystem
  u-sub : Subsystem
  v-sub : Subsystem
  u : Outport
  v : Outport  Port=2
  r : Outport  Port=3
  x : Outport  Port=4
  y : Outport  Port=5
  ψ : Outport  Port=6
  wires:
  m/1 -> v-sub/2(m), u-sub/2(m)
  Y/1 -> v-sub/1(Y)
  r-sub/1(r) -> r/1, u-sub/6(r), v-sub/6(r), Integrator2/1
  Izz/1 -> r-sub/2(Izz)
  N/1 -> r-sub/1(N)
  Jzz/1 -> r-sub/3(Jzz)
  X/1 -> u-sub/1(X)
  my/1 -> u-sub/3(my), v-sub/4(my)
  mx/1 -> u-sub/4(mx), v-sub/3(mx)
  v-sub/1(v) -> dy/2(v), dx/2(v), v/1, u-sub/5(v)
  u-sub/1(u) -> u/1, dy/1(u), dx/1(u), v-sub/5(u)
  dy/1(dy) -> Integrator3/1
  dx/1(dx) -> Integrator1/1
  Integrator3/1 -> y/1
  Integrator1/1 -> x/1
  Gain/1 -> ψ/1
  Integrator2/1 -> Gain/1, dy/3(fai), dx/3(fai)

== system MASs_cp/usv3/USV/F model ==
  n : Inport
  δ : Inport  Port=2
  u : Inport  Port=3
  v : Inport  Port=4
  r : Inport  Port=5
  Add : Sum  Inputs=3
  Add1 : Sum  Inputs=3
  Add2 : Sum  Inputs=3
  P model : Subsystem
  S model : Subsystem
  W model : Subsystem
  X : Outport
  Y : Outport  Port=2
  N : Outport  Port=3
  wires:
  n/1 -> P model/1(n)
  δ/1 -> P model/2(δ)
  P model/1(Xp) -> Add/1
  W model/1(Xw) -> Add/2
  S model/1(Xs) -> Add/3
  P model/2(Yp) -> Add1/1
  W model/2(Yw) -> Add1/2
  S model/2(Ys) -> Add1/3
  P model/3(Np) -> Add2/1
  W model/3(Nw) -> Add2/2
  S model/3(Ns) -> Add2/3
  Add/1 -> X/1
  Add1/1 -> Y/1
  Add2/1 -> N/1
  u/1 -> S model/1(u), P model/3(u)
  v/1 -> S model/2(v), P model/4(v)
  r/1 -> S model/3(r)

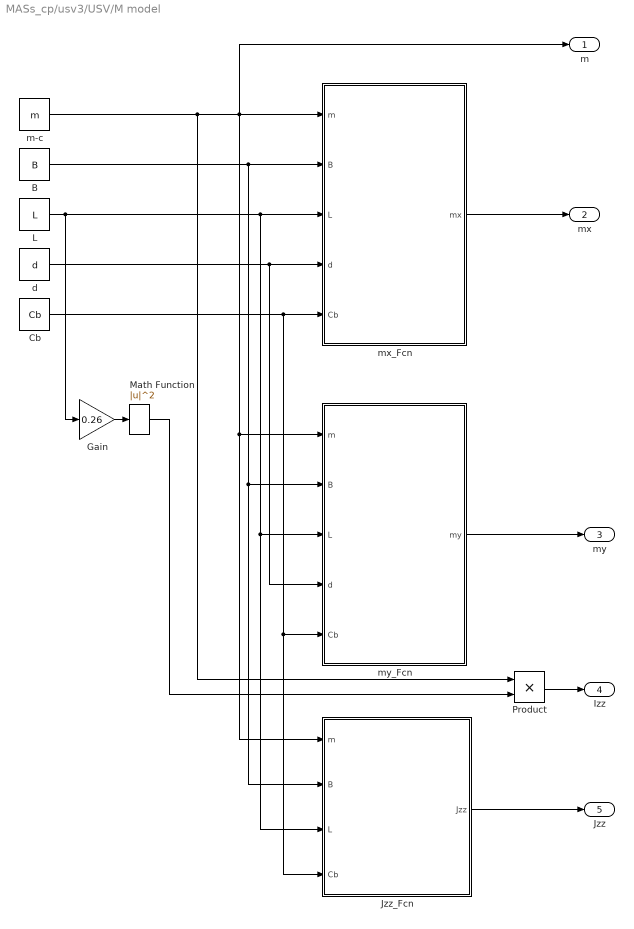
== system MASs_cp/usv3/USV/M model ==
  B : Constant  Value=B
  Cb : Constant  Value=Cb
  Gain : Gain  Gain=0.26
  Jzz_Fcn : MATLAB Function  TreatAsAtomicUnit=on
  L : Constant  Value=L
  Math Function : Math  Operator=magnitude^2  SaturateOnIntegerOverflow=on
  Product : Product
  d : Constant  Value=d
  m-c : Constant  Value=m
  mx_Fcn : MATLAB Function  TreatAsAtomicUnit=on
  my_Fcn : MATLAB Function  TreatAsAtomicUnit=on
  m : Outport
  mx : Outport  Port=2
  my : Outport  Port=3
  Izz : Outport  Port=4
  Jzz : Outport  Port=5
  wires:
  mx_Fcn/1(mx) -> mx/1
  d/1 -> my_Fcn/4(d), mx_Fcn/4(d)
  B/1 -> Jzz_Fcn/2(B), my_Fcn/2(B), mx_Fcn/2(B)
  my_Fcn/1(my) -> my/1
  Jzz_Fcn/1(Jzz) -> Jzz/1
  m-c/1 -> Product/1, m/1, Jzz_Fcn/1(m), my_Fcn/1(m), mx_Fcn/1(m)
  L/1 -> Gain/1, Jzz_Fcn/3(L), my_Fcn/3(L), mx_Fcn/3(L)
  Cb/1 -> Jzz_Fcn/4(Cb), my_Fcn/5(Cb), mx_Fcn/5(Cb)
  Gain/1 -> Math Function/1
  Product/1 -> Izz/1
  Math Function/1 -> Product/2

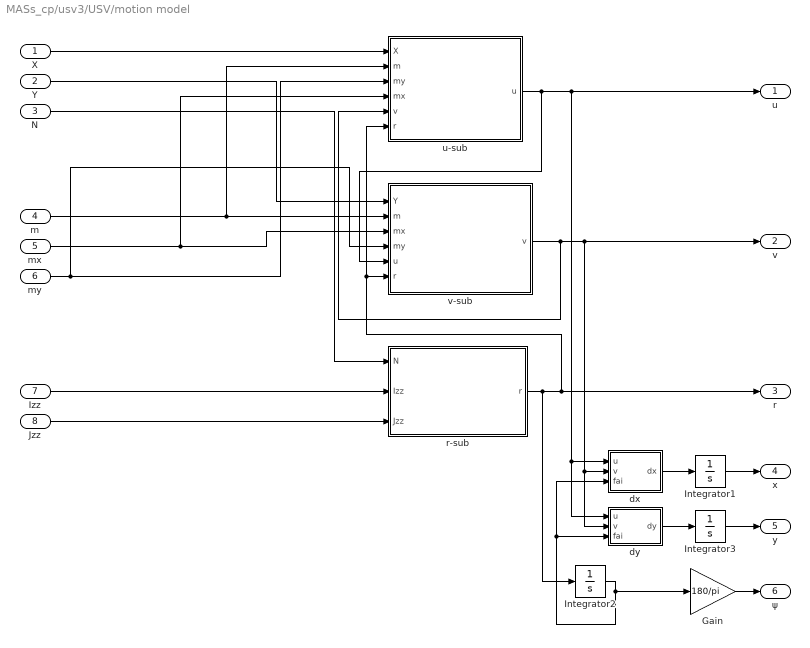
== system MASs_cp/usv3/USV/motion model ==
  X : Inport
  Y : Inport  Port=2
  N : Inport  Port=3
  m : Inport  Port=4
  mx : Inport  Port=5
  my : Inport  Port=6
  Izz : Inport  Port=7
  Jzz : Inport  Port=8
  Gain : Gain  Gain=180/pi
  Integrator1 : Integrator
  Integrator2 : Integrator  InitialCondition=rand()*pi-pi/2
  Integrator3 : Integrator
  dx : MATLAB Function  TreatAsAtomicUnit=on
  dy : MATLAB Function  TreatAsAtomicUnit=on
  r-sub : Subsystem
  u-sub : Subsystem
  v-sub : Subsystem
  u : Outport
  v : Outport  Port=2
  r : Outport  Port=3
  x : Outport  Port=4
  y : Outport  Port=5
  ψ : Outport  Port=6
  wires:
  m/1 -> v-sub/2(m), u-sub/2(m)
  Y/1 -> v-sub/1(Y)
  r-sub/1(r) -> r/1, u-sub/6(r), v-sub/6(r), Integrator2/1
  Izz/1 -> r-sub/2(Izz)
  N/1 -> r-sub/1(N)
  Jzz/1 -> r-sub/3(Jzz)
  X/1 -> u-sub/1(X)
  my/1 -> u-sub/3(my), v-sub/4(my)
  mx/1 -> u-sub/4(mx), v-sub/3(mx)
  v-sub/1(v) -> dy/2(v), dx/2(v), v/1, u-sub/5(v)
  u-sub/1(u) -> u/1, dy/1(u), dx/1(u), v-sub/5(u)
  dy/1(dy) -> Integrator3/1
  dx/1(dx) -> Integrator1/1
  Integrator3/1 -> y/1
  Integrator1/1 -> x/1
  Gain/1 -> ψ/1
  Integrator2/1 -> Gain/1, dy/3(fai), dx/3(fai)

== system MASs_cp/usv4/USV/F model ==
  n : Inport
  δ : Inport  Port=2
  u : Inport  Port=3
  v : Inport  Port=4
  r : Inport  Port=5
  Add : Sum  Inputs=3
  Add1 : Sum  Inputs=3
  Add2 : Sum  Inputs=3
  P model : Subsystem
  S model : Subsystem
  W model : Subsystem
  X : Outport
  Y : Outport  Port=2
  N : Outport  Port=3
  wires:
  n/1 -> P model/1(n)
  δ/1 -> P model/2(δ)
  P model/1(Xp) -> Add/1
  W model/1(Xw) -> Add/2
  S model/1(Xs) -> Add/3
  P model/2(Yp) -> Add1/1
  W model/2(Yw) -> Add1/2
  S model/2(Ys) -> Add1/3
  P model/3(Np) -> Add2/1
  W model/3(Nw) -> Add2/2
  S model/3(Ns) -> Add2/3
  Add/1 -> X/1
  Add1/1 -> Y/1
  Add2/1 -> N/1
  u/1 -> S model/1(u), P model/3(u)
  v/1 -> S model/2(v), P model/4(v)
  r/1 -> S model/3(r)

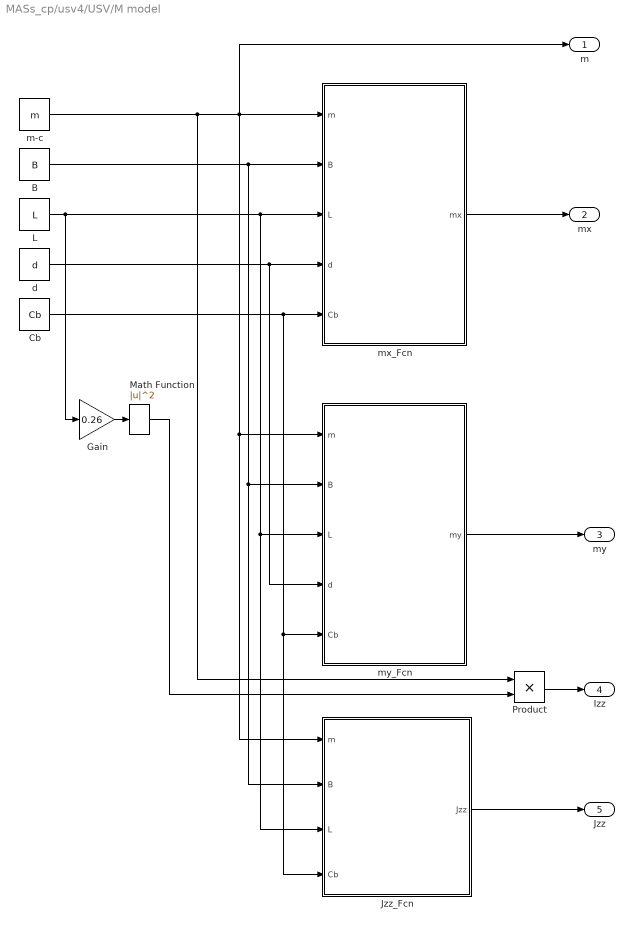
== system MASs_cp/usv4/USV/M model ==
  B : Constant  Value=B
  Cb : Constant  Value=Cb
  Gain : Gain  Gain=0.26
  Jzz_Fcn : MATLAB Function  TreatAsAtomicUnit=on
  L : Constant  Value=L
  Math Function : Math  Operator=magnitude^2  SaturateOnIntegerOverflow=on
  Product : Product
  d : Constant  Value=d
  m-c : Constant  Value=m
  mx_Fcn : MATLAB Function  TreatAsAtomicUnit=on
  my_Fcn : MATLAB Function  TreatAsAtomicUnit=on
  m : Outport
  mx : Outport  Port=2
  my : Outport  Port=3
  Izz : Outport  Port=4
  Jzz : Outport  Port=5
  wires:
  mx_Fcn/1(mx) -> mx/1
  d/1 -> my_Fcn/4(d), mx_Fcn/4(d)
  B/1 -> Jzz_Fcn/2(B), my_Fcn/2(B), mx_Fcn/2(B)
  my_Fcn/1(my) -> my/1
  Jzz_Fcn/1(Jzz) -> Jzz/1
  m-c/1 -> Product/1, m/1, Jzz_Fcn/1(m), my_Fcn/1(m), mx_Fcn/1(m)
  L/1 -> Gain/1, Jzz_Fcn/3(L), my_Fcn/3(L), mx_Fcn/3(L)
  Cb/1 -> Jzz_Fcn/4(Cb), my_Fcn/5(Cb), mx_Fcn/5(Cb)
  Gain/1 -> Math Function/1
  Product/1 -> Izz/1
  Math Function/1 -> Product/2

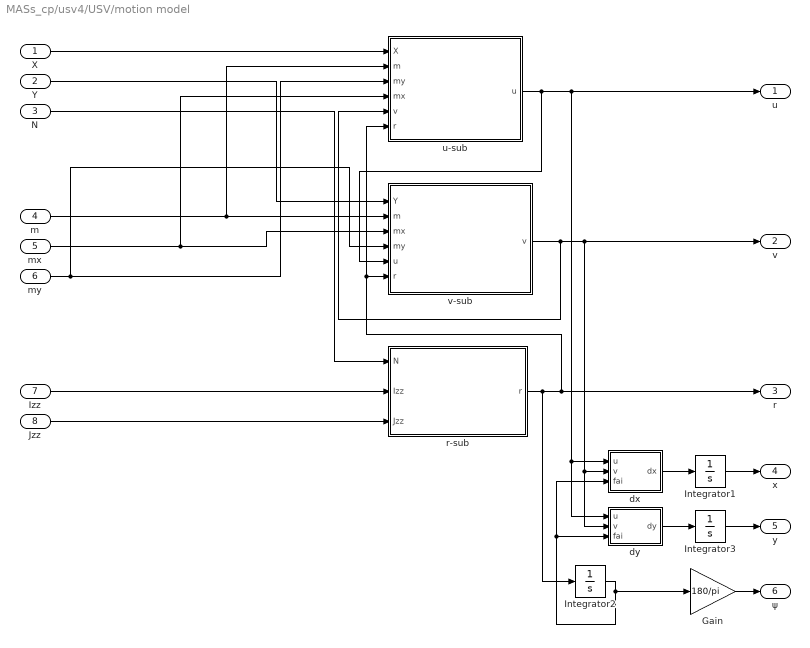
== system MASs_cp/usv4/USV/motion model ==
  X : Inport
  Y : Inport  Port=2
  N : Inport  Port=3
  m : Inport  Port=4
  mx : Inport  Port=5
  my : Inport  Port=6
  Izz : Inport  Port=7
  Jzz : Inport  Port=8
  Gain : Gain  Gain=180/pi
  Integrator1 : Integrator
  Integrator2 : Integrator  InitialCondition=rand()*pi-pi/2
  Integrator3 : Integrator
  dx : MATLAB Function  TreatAsAtomicUnit=on
  dy : MATLAB Function  TreatAsAtomicUnit=on
  r-sub : Subsystem
  u-sub : Subsystem
  v-sub : Subsystem
  u : Outport
  v : Outport  Port=2
  r : Outport  Port=3
  x : Outport  Port=4
  y : Outport  Port=5
  ψ : Outport  Port=6
  wires:
  m/1 -> v-sub/2(m), u-sub/2(m)
  Y/1 -> v-sub/1(Y)
  r-sub/1(r) -> r/1, u-sub/6(r), v-sub/6(r), Integrator2/1
  Izz/1 -> r-sub/2(Izz)
  N/1 -> r-sub/1(N)
  Jzz/1 -> r-sub/3(Jzz)
  X/1 -> u-sub/1(X)
  my/1 -> u-sub/3(my), v-sub/4(my)
  mx/1 -> u-sub/4(mx), v-sub/3(mx)
  v-sub/1(v) -> dy/2(v), dx/2(v), v/1, u-sub/5(v)
  u-sub/1(u) -> u/1, dy/1(u), dx/1(u), v-sub/5(u)
  dy/1(dy) -> Integrator3/1
  dx/1(dx) -> Integrator1/1
  Integrator3/1 -> y/1
  Integrator1/1 -> x/1
  Gain/1 -> ψ/1
  Integrator2/1 -> Gain/1, dy/3(fai), dx/3(fai)

== system MASs_cp/usv5/USV/F model ==
  n : Inport
  δ : Inport  Port=2
  u : Inport  Port=3
  v : Inport  Port=4
  r : Inport  Port=5
  Add : Sum  Inputs=3
  Add1 : Sum  Inputs=3
  Add2 : Sum  Inputs=3
  P model : Subsystem
  S model : Subsystem
  W model : Subsystem
  X : Outport
  Y : Outport  Port=2
  N : Outport  Port=3
  wires:
  n/1 -> P model/1(n)
  δ/1 -> P model/2(δ)
  P model/1(Xp) -> Add/1
  W model/1(Xw) -> Add/2
  S model/1(Xs) -> Add/3
  P model/2(Yp) -> Add1/1
  W model/2(Yw) -> Add1/2
  S model/2(Ys) -> Add1/3
  P model/3(Np) -> Add2/1
  W model/3(Nw) -> Add2/2
  S model/3(Ns) -> Add2/3
  Add/1 -> X/1
  Add1/1 -> Y/1
  Add2/1 -> N/1
  u/1 -> S model/1(u), P model/3(u)
  v/1 -> S model/2(v), P model/4(v)
  r/1 -> S model/3(r)

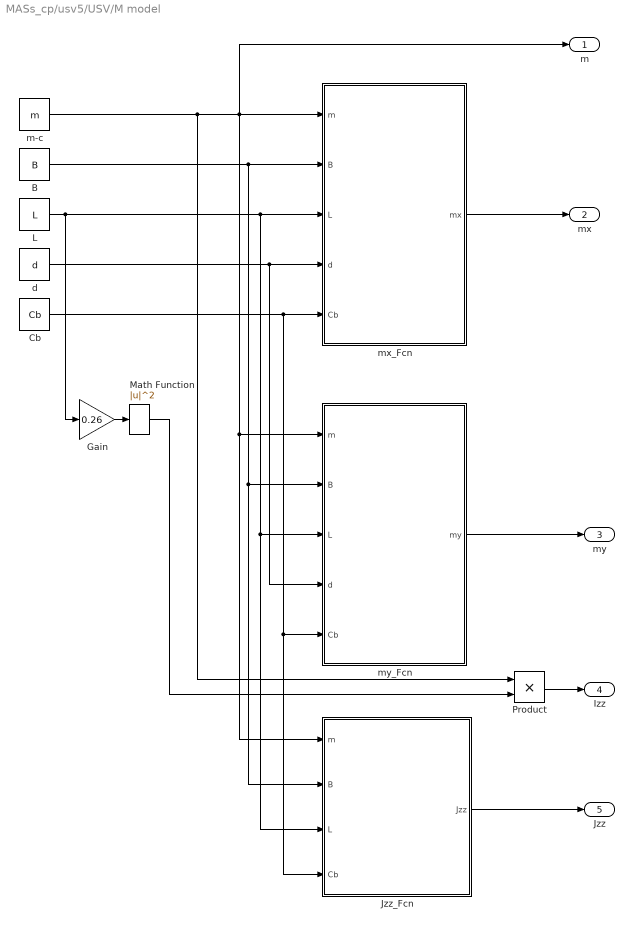
== system MASs_cp/usv5/USV/M model ==
  B : Constant  Value=B
  Cb : Constant  Value=Cb
  Gain : Gain  Gain=0.26
  Jzz_Fcn : MATLAB Function  TreatAsAtomicUnit=on
  L : Constant  Value=L
  Math Function : Math  Operator=magnitude^2  SaturateOnIntegerOverflow=on
  Product : Product
  d : Constant  Value=d
  m-c : Constant  Value=m
  mx_Fcn : MATLAB Function  TreatAsAtomicUnit=on
  my_Fcn : MATLAB Function  TreatAsAtomicUnit=on
  m : Outport
  mx : Outport  Port=2
  my : Outport  Port=3
  Izz : Outport  Port=4
  Jzz : Outport  Port=5
  wires:
  mx_Fcn/1(mx) -> mx/1
  d/1 -> my_Fcn/4(d), mx_Fcn/4(d)
  B/1 -> Jzz_Fcn/2(B), my_Fcn/2(B), mx_Fcn/2(B)
  my_Fcn/1(my) -> my/1
  Jzz_Fcn/1(Jzz) -> Jzz/1
  m-c/1 -> Product/1, m/1, Jzz_Fcn/1(m), my_Fcn/1(m), mx_Fcn/1(m)
  L/1 -> Gain/1, Jzz_Fcn/3(L), my_Fcn/3(L), mx_Fcn/3(L)
  Cb/1 -> Jzz_Fcn/4(Cb), my_Fcn/5(Cb), mx_Fcn/5(Cb)
  Gain/1 -> Math Function/1
  Product/1 -> Izz/1
  Math Function/1 -> Product/2

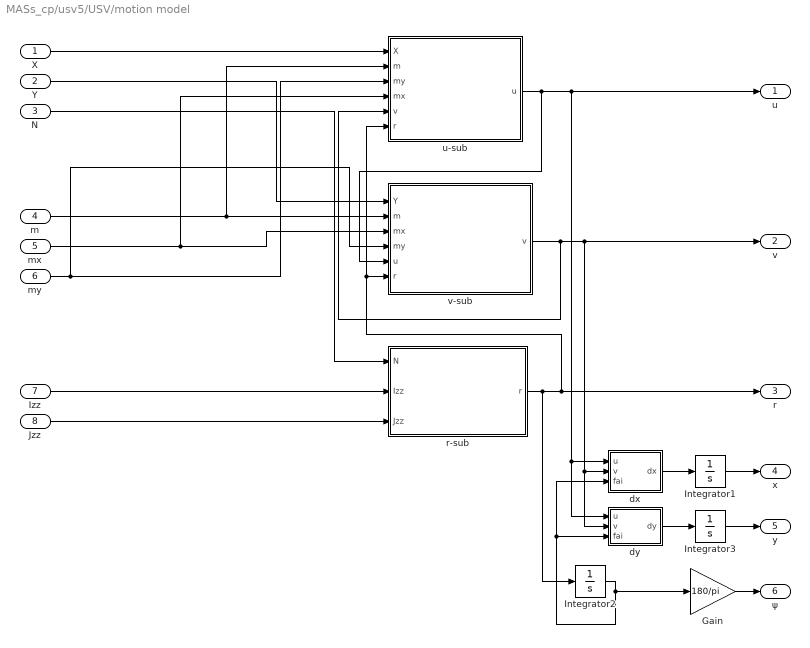
== system MASs_cp/usv5/USV/motion model ==
  X : Inport
  Y : Inport  Port=2
  N : Inport  Port=3
  m : Inport  Port=4
  mx : Inport  Port=5
  my : Inport  Port=6
  Izz : Inport  Port=7
  Jzz : Inport  Port=8
  Gain : Gain  Gain=180/pi
  Integrator1 : Integrator
  Integrator2 : Integrator  InitialCondition=rand()*pi-pi/2
  Integrator3 : Integrator
  dx : MATLAB Function  TreatAsAtomicUnit=on
  dy : MATLAB Function  TreatAsAtomicUnit=on
  r-sub : Subsystem
  u-sub : Subsystem
  v-sub : Subsystem
  u : Outport
  v : Outport  Port=2
  r : Outport  Port=3
  x : Outport  Port=4
  y : Outport  Port=5
  ψ : Outport  Port=6
  wires:
  m/1 -> v-sub/2(m), u-sub/2(m)
  Y/1 -> v-sub/1(Y)
  r-sub/1(r) -> r/1, u-sub/6(r), v-sub/6(r), Integrator2/1
  Izz/1 -> r-sub/2(Izz)
  N/1 -> r-sub/1(N)
  Jzz/1 -> r-sub/3(Jzz)
  X/1 -> u-sub/1(X)
  my/1 -> u-sub/3(my), v-sub/4(my)
  mx/1 -> u-sub/4(mx), v-sub/3(mx)
  v-sub/1(v) -> dy/2(v), dx/2(v), v/1, u-sub/5(v)
  u-sub/1(u) -> u/1, dy/1(u), dx/1(u), v-sub/5(u)
  dy/1(dy) -> Integrator3/1
  dx/1(dx) -> Integrator1/1
  Integrator3/1 -> y/1
  Integrator1/1 -> x/1
  Gain/1 -> ψ/1
  Integrator2/1 -> Gain/1, dy/3(fai), dx/3(fai)

== system MASs_cp/usv1/USV/F model/P model ==
  n : Inport
  δ : Inport  Port=2
  u : Inport  Port=3
  v : Inport  Port=4
  p-fcn : MATLAB Function  TreatAsAtomicUnit=on
  Xp : Outport
  Yp : Outport  Port=2
  Np : Outport  Port=3
  wires:
  p-fcn/3(Np) -> Np/1
  p-fcn/2(Yp) -> Yp/1
  p-fcn/1(Xp) -> Xp/1
  n/1 -> p-fcn/1(n)
  δ/1 -> p-fcn/2(sita)
  u/1 -> p-fcn/3(u)
  v/1 -> p-fcn/4(v)

== system MASs_cp/usv1/USV/F model/S model ==
  u : Inport
  v : Inport  Port=2
  r : Inport  Port=3
  B : Constant  Value=B
  Cb : Constant  Value=Cb
  L : Constant  Value=L
  d : Constant  Value=d
  m : Constant  Value=m
  s-fcn : MATLAB Function  TreatAsAtomicUnit=on
  Xs : Outport
  Ys : Outport  Port=2
  Ns : Outport  Port=3
  wires:
  s-fcn/1(Xs) -> Xs/1
  s-fcn/2(Ys) -> Ys/1
  s-fcn/3(Ns) -> Ns/1
  B/1 -> s-fcn/1(B)
  d/1 -> s-fcn/2(d)
  L/1 -> s-fcn/3(L)
  u/1 -> s-fcn/6(u)
  v/1 -> s-fcn/7(v)
  r/1 -> s-fcn/8(r)
  Cb/1 -> s-fcn/4(Cb)
  m/1 -> s-fcn/5(m)

== system MASs_cp/usv1/USV/F model/W model ==
  n : Constant  Value=0
  n1 : Constant  Value=0
  n2 : Constant  Value=0
  Xw : Outport
  Yw : Outport  Port=2
  Nw : Outport  Port=3
  wires:
  n/1 -> Xw/1
  n2/1 -> Yw/1
  n1/1 -> Nw/1

== system MASs_cp/usv1/USV/motion model/r-sub ==
  N : Inport
  Izz : Inport  Port=2
  Jzz : Inport  Port=3
  Divide2 : Product  Inputs=*/
  Integrator2 : Integrator
  Sum4 : Sum  Inputs=|++
  r : Outport
  wires:
  Sum4/1 -> Divide2/2
  Divide2/1 -> Integrator2/1  "r'"
  Integrator2/1 -> r/1  "r"
  N/1 -> Divide2/1
  Jzz/1 -> Sum4/2
  Izz/1 -> Sum4/1

== system MASs_cp/usv1/USV/motion model/u-sub ==
  X : Inport
  m : Inport  Port=2
  my : Inport  Port=3
  mx : Inport  Port=4
  v : Inport  Port=5
  r : Inport  Port=6
  Add : Sum
  Divide1 : Product  Inputs=*/
  Integrator : Integrator
  Product : Product  Inputs=3
  Sum : Sum  Inputs=|++
  Sum1 : Sum  Inputs=|++
  u : Outport
  wires:
  Sum1/1 -> Divide1/2
  Divide1/1 -> Integrator/1  "u'"
  Integrator/1 -> u/1  "u"
  Sum/1 -> Product/1
  Add/1 -> Divide1/1
  my/1 -> Sum/2
  X/1 -> Add/1
  v/1 -> Product/2
  r/1 -> Product/3
  mx/1 -> Sum1/2
  m/1 -> Sum1/1, Sum/1
  Product/1 -> Add/2

== system MASs_cp/usv1/USV/motion model/v-sub ==
  Y : Inport
  m : Inport  Port=2
  mx : Inport  Port=3
  my : Inport  Port=4
  u : Inport  Port=5
  r : Inport  Port=6
  Add2 : Sum  Inputs=+-
  Divide3 : Product  Inputs=*/
  Integrator1 : Integrator
  Product1 : Product  Inputs=3
  Sum2 : Sum  Inputs=|++
  Sum3 : Sum  Inputs=|++
  v : Outport
  wires:
  Sum3/1 -> Divide3/2
  my/1 -> Sum3/1
  r/1 -> Product1/3
  Product1/1 -> Add2/2
  m/1 -> Sum3/2, Sum2/1
  Sum2/1 -> Product1/1
  Y/1 -> Add2/1
  Add2/1 -> Divide3/1
  Divide3/1 -> Integrator1/1  "v'"
  Integrator1/1 -> v/1  "v"
  u/1 -> Product1/2
  mx/1 -> Sum2/2

== system MASs_cp/usv2/USV/F model/P model ==
  n : Inport
  δ : Inport  Port=2
  u : Inport  Port=3
  v : Inport  Port=4
  p-fcn : MATLAB Function  TreatAsAtomicUnit=on
  Xp : Outport
  Yp : Outport  Port=2
  Np : Outport  Port=3
  wires:
  p-fcn/3(Np) -> Np/1
  p-fcn/2(Yp) -> Yp/1
  p-fcn/1(Xp) -> Xp/1
  n/1 -> p-fcn/1(n)
  δ/1 -> p-fcn/2(sita)
  u/1 -> p-fcn/3(u)
  v/1 -> p-fcn/4(v)

== system MASs_cp/usv2/USV/F model/S model ==
  u : Inport
  v : Inport  Port=2
  r : Inport  Port=3
  B : Constant  Value=B
  Cb : Constant  Value=Cb
  L : Constant  Value=L
  d : Constant  Value=d
  m : Constant  Value=m
  s-fcn : MATLAB Function  TreatAsAtomicUnit=on
  Xs : Outport
  Ys : Outport  Port=2
  Ns : Outport  Port=3
  wires:
  s-fcn/1(Xs) -> Xs/1
  s-fcn/2(Ys) -> Ys/1
  s-fcn/3(Ns) -> Ns/1
  B/1 -> s-fcn/1(B)
  d/1 -> s-fcn/2(d)
  L/1 -> s-fcn/3(L)
  u/1 -> s-fcn/6(u)
  v/1 -> s-fcn/7(v)
  r/1 -> s-fcn/8(r)
  Cb/1 -> s-fcn/4(Cb)
  m/1 -> s-fcn/5(m)

== system MASs_cp/usv2/USV/F model/W model ==
  n : Constant  Value=0
  n1 : Constant  Value=0
  n2 : Constant  Value=0
  Xw : Outport
  Yw : Outport  Port=2
  Nw : Outport  Port=3
  wires:
  n/1 -> Xw/1
  n2/1 -> Yw/1
  n1/1 -> Nw/1

== system MASs_cp/usv2/USV/motion model/r-sub ==
  N : Inport
  Izz : Inport  Port=2
  Jzz : Inport  Port=3
  Divide2 : Product  Inputs=*/
  Integrator2 : Integrator
  Sum4 : Sum  Inputs=|++
  r : Outport
  wires:
  Sum4/1 -> Divide2/2
  Divide2/1 -> Integrator2/1  "r'"
  Integrator2/1 -> r/1  "r"
  N/1 -> Divide2/1
  Jzz/1 -> Sum4/2
  Izz/1 -> Sum4/1

== system MASs_cp/usv2/USV/motion model/u-sub ==
  X : Inport
  m : Inport  Port=2
  my : Inport  Port=3
  mx : Inport  Port=4
  v : Inport  Port=5
  r : Inport  Port=6
  Add : Sum
  Divide1 : Product  Inputs=*/
  Integrator : Integrator
  Product : Product  Inputs=3
  Sum : Sum  Inputs=|++
  Sum1 : Sum  Inputs=|++
  u : Outport
  wires:
  Sum1/1 -> Divide1/2
  Divide1/1 -> Integrator/1  "u'"
  Integrator/1 -> u/1  "u"
  Sum/1 -> Product/1
  Add/1 -> Divide1/1
  my/1 -> Sum/2
  X/1 -> Add/1
  v/1 -> Product/2
  r/1 -> Product/3
  mx/1 -> Sum1/2
  m/1 -> Sum1/1, Sum/1
  Product/1 -> Add/2

== system MASs_cp/usv2/USV/motion model/v-sub ==
  Y : Inport
  m : Inport  Port=2
  mx : Inport  Port=3
  my : Inport  Port=4
  u : Inport  Port=5
  r : Inport  Port=6
  Add2 : Sum  Inputs=+-
  Divide3 : Product  Inputs=*/
  Integrator1 : Integrator
  Product1 : Product  Inputs=3
  Sum2 : Sum  Inputs=|++
  Sum3 : Sum  Inputs=|++
  v : Outport
  wires:
  Sum3/1 -> Divide3/2
  my/1 -> Sum3/1
  r/1 -> Product1/3
  Product1/1 -> Add2/2
  m/1 -> Sum3/2, Sum2/1
  Sum2/1 -> Product1/1
  Y/1 -> Add2/1
  Add2/1 -> Divide3/1
  Divide3/1 -> Integrator1/1  "v'"
  Integrator1/1 -> v/1  "v"
  u/1 -> Product1/2
  mx/1 -> Sum2/2

== system MASs_cp/usv3/USV/F model/P model ==
  n : Inport
  δ : Inport  Port=2
  u : Inport  Port=3
  v : Inport  Port=4
  p-fcn : MATLAB Function  TreatAsAtomicUnit=on
  Xp : Outport
  Yp : Outport  Port=2
  Np : Outport  Port=3
  wires:
  p-fcn/3(Np) -> Np/1
  p-fcn/2(Yp) -> Yp/1
  p-fcn/1(Xp) -> Xp/1
  n/1 -> p-fcn/1(n)
  δ/1 -> p-fcn/2(sita)
  u/1 -> p-fcn/3(u)
  v/1 -> p-fcn/4(v)
